simulink model "DiagramaDeSimulacaoItem3"  (R2019a)
settings: Solver=VariableStepAuto  StartTime=0.0  StopTime=5  RelTol=1e-3
undefined symbols (not defined in the file): CaEq, CafEq, k1, k2, k3, uEq
settings Model: Creator=Usuario  LastModifiedBy=Usuario

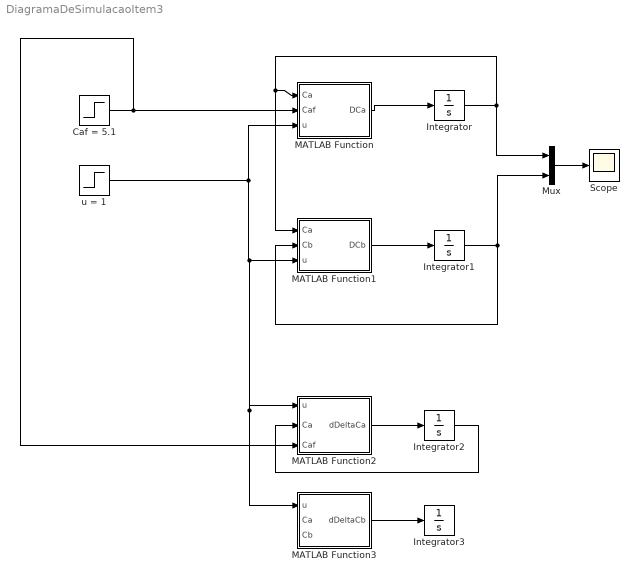
== system DiagramaDeSimulacaoItem3 ==
  Caf = 5.1 : Step  Time=0  After=5.1  SampleTime=0
  Integrator{,1..3} (4 alike) : Integrator
  MATLAB Function : MATLAB Function  TreatAsAtomicUnit=on
  MATLAB Function1 : MATLAB Function  TreatAsAtomicUnit=on
  MATLAB Function2 : MATLAB Function  TreatAsAtomicUnit=on
  MATLAB Function3 : MATLAB Function  TreatAsAtomicUnit=on
  Mux : Mux  Inputs=2
  Scope : Scope
  "u = 1 " : Step  Time=0  SampleTime=0
  wires:
  MATLAB Function/1(DCa) -> Integrator/1
  MATLAB Function1/1(DCb) -> Integrator1/1
  Integrator/1 -> Mux/1, MATLAB Function1/1(Ca), MATLAB Function/1(Ca)
  Integrator1/1 -> MATLAB Function1/2(Cb), Mux/2
  Mux/1 -> Scope/1
  "u = 1 "/1 -> MATLAB Function/3(u), MATLAB Function3/1(u), MATLAB Function2/1(u), MATLAB Function1/3(u)
  Caf = 5.1/1 -> MATLAB Function/2(Caf), MATLAB Function2/3(Caf)
  MATLAB Function2/1(dDeltaCa) -> Integrator2/1
  MATLAB Function3/1(dDeltaCb) -> Integrator3/1
  Integrator2/1 -> MATLAB Function2/2(Ca)

== matlab function DiagramaDeSimulacaoItem3/MATLAB Function1 ==
  data: DCb output; Ca input; Cb input; u input; k2 parameter; k1 parameter
function DCb = fcn(Ca,Cb,u, k2, k1)

DCb = k1*Ca - k2*Cb - Cb*u;

== matlab function DiagramaDeSimulacaoItem3/MATLAB Function ==
  data: DCa output; Ca input; Caf input; k1 parameter; k3 parameter; u input
function DCa = fcn(Ca,Caf,k1, k3, u)

DCa = -k1*Ca - k3*Ca^2 + (Caf -Ca)*u;

== matlab function DiagramaDeSimulacaoItem3/MATLAB Function2 ==
  data: u input; dDeltaCa output; Ca input; Caf input; CaEq parameter; k1 parameter; k3 parameter; uEq parameter; CafEq parameter
function dDeltaCa = fcn(u,Ca,Caf, CaEq, k1, k3, uEq, CafEq)

dDeltaCa = (Ca-CaEq)*(-k1-2*k3*CaEq - uEq) + (u-uEq)*(CafEq-CaEq) + (Caf-CafEq)*uEq;

== matlab function DiagramaDeSimulacaoItem3/MATLAB Function3 ==
  data: u input; dDeltaCb output; Ca input; CaEq parameter; k1 parameter; k2 parameter; uEq parameter; Cb input
function dDeltaCb = fcn(u,Ca, CaEq, k1, k2, uEq, Cb)

dDeltaCb = (Ca-CaEq)*(k1) + (Cb-CbEq)*(-uEq-k2) + (u-uEq)*(-CbEq);
